simulink model "BumplessPID_UuT_Harness1"  (R2020a)
settings: Solver=ode8  StartTime=0.0  StopTime=40  FixedStep=0.1  RelTol=1e-3
settings Model: PauseTimes=12  Creator=Christian  LastModifiedBy=Christian

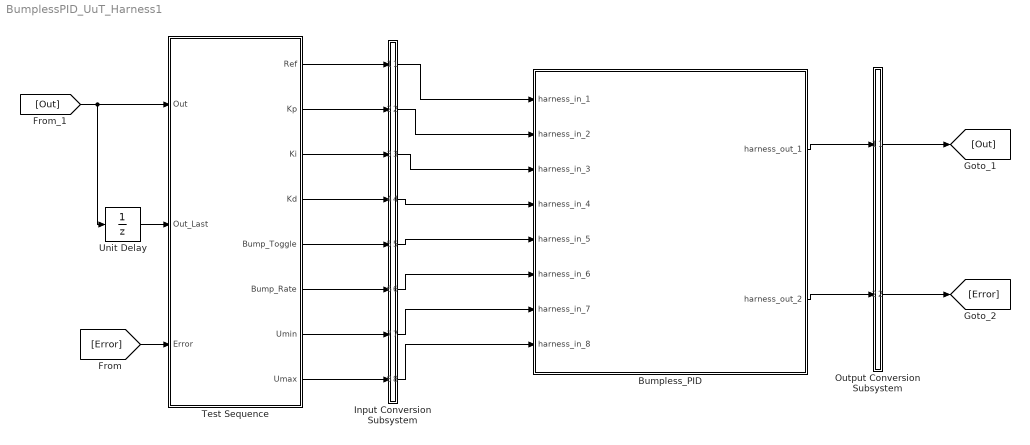
== system BumplessPID_UuT_Harness1 ==
  Bumpless_PID : Subsystem  Tag=__SL_testing_harness_stub_
  Input Conversion Subsystem : Subsystem  Tag=__SLT_ICS__  Description=|
      | Signal spec.
      | and routing
      settings: AttributesFormatString=%<Description>
  Output Conversion Subsystem : Subsystem  Tag=__SLT_OCS__  Description=|
      | Signal spec.
      | and routing
      settings: AttributesFormatString=%<Description>
  Test Sequence : Test Sequence  TreatAsAtomicUnit=on
  Unit Delay : UnitDelay  SampleTime=-1  HasFrameUpgradeWarning=on
  wires:
  Test Sequence/1(Ref) -> Input Conversion Subsystem/1(Inport_1)
  Test Sequence/2(Kp) -> Input Conversion Subsystem/2(Inport_2)
  Test Sequence/3(Ki) -> Input Conversion Subsystem/3(Inport_3)
  Test Sequence/4(Kd) -> Input Conversion Subsystem/4(Inport_4)
  Test Sequence/5(Bump_Toggle) -> Input Conversion Subsystem/5(Inport_5)
  Test Sequence/6(Bump_Rate) -> Input Conversion Subsystem/6(Inport_6)
  [Out] -> Unit Delay/1, Test Sequence/1(Out)
  Output Conversion Subsystem/1(Outport_1) -> [Out]
  Output Conversion Subsystem/2(Outport_2) -> [Error]
  [Error] -> Test Sequence/3(Error)
  Bumpless_PID/1(harness_out_1) -> Output Conversion Subsystem/1(Inport_1)
  Bumpless_PID/2(harness_out_2) -> Output Conversion Subsystem/2(Inport_2)
  Input Conversion Subsystem/1(Outport_1) -> Bumpless_PID/1(harness_in_1)
  Input Conversion Subsystem/2(Outport_2) -> Bumpless_PID/2(harness_in_2)
  Input Conversion Subsystem/3(Outport_3) -> Bumpless_PID/3(harness_in_3)
  Input Conversion Subsystem/4(Outport_4) -> Bumpless_PID/4(harness_in_4)
  Input Conversion Subsystem/5(Outport_5) -> Bumpless_PID/5(harness_in_5)
  Input Conversion Subsystem/6(Outport_6) -> Bumpless_PID/6(harness_in_6)
  Input Conversion Subsystem/7(Outport_7) -> Bumpless_PID/7(harness_in_7)
  Input Conversion Subsystem/8(Outport_8) -> Bumpless_PID/8(harness_in_8)
  Test Sequence/7(Umin) -> Input Conversion Subsystem/7(Inport_7)
  Test Sequence/8(Umax) -> Input Conversion Subsystem/8(Inport_8)
  Unit Delay/1 -> Test Sequence/2(Out_Last)

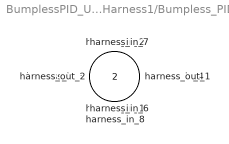
== system BumplessPID_UuT_Harness1/Bumpless_PID ==
  harness_in_1 : Inport
  harness_in_2 : Inport  Port=2
  harness_in_3 : Inport  Port=3
  harness_in_4 : Inport  Port=4
  harness_in_5 : Inport  Port=5
  harness_in_6 : Inport  Port=6
  harness_in_7 : Inport  Port=7
  harness_in_8 : Inport  Port=8
  harness_out_1 : Outport
  harness_out_2 : Outport  Port=2

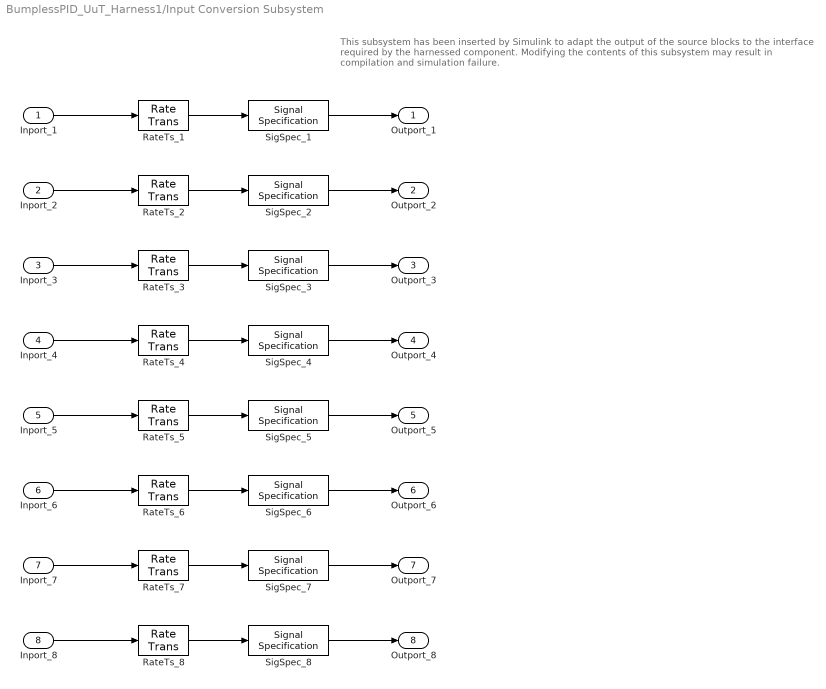
== system BumplessPID_UuT_Harness1/Input Conversion Subsystem ==
  note: This subsystem has been inserted by Simulink to adapt the output of the source blocks to the interface required by the harnessed component.
      |  Modifying the contents of this subsystem may result in compilation and simulation failure.
  Inport_1 : Inport
  Inport_2 : Inport  Port=2
  Inport_3 : Inport  Port=3
  Inport_4 : Inport  Port=4
  Inport_5 : Inport  Port=5
  Inport_6 : Inport  Port=6
  Inport_7 : Inport  Port=7
  Inport_8 : Inport  Port=8
  RateTs_{1..8} (8 alike) : RateTransition  OutPortSampleTime=[-1, 0]
  SigSpec_{1..6} (6 alike) : SignalSpecification  OutDataTypeStr=double  Dimensions=[1]  SampleTime=[-1, 0]
  SigSpec_7 : SignalSpecification  OutDataTypeStr=double  Dimensions=[1]
  SigSpec_8 : SignalSpecification  OutDataTypeStr=double  Dimensions=[1]
  Outport_1 : Outport
  Outport_2 : Outport  Port=2
  Outport_3 : Outport  Port=3
  Outport_4 : Outport  Port=4
  Outport_5 : Outport  Port=5
  Outport_6 : Outport  Port=6
  Outport_7 : Outport  Port=7
  Outport_8 : Outport  Port=8
  wires:
  SigSpec_1/1 -> Outport_1/1
  RateTs_1/1 -> SigSpec_1/1
  Inport_1/1 -> RateTs_1/1
  SigSpec_2/1 -> Outport_2/1
  RateTs_2/1 -> SigSpec_2/1
  Inport_2/1 -> RateTs_2/1
  SigSpec_3/1 -> Outport_3/1
  RateTs_3/1 -> SigSpec_3/1
  Inport_3/1 -> RateTs_3/1
  SigSpec_4/1 -> Outport_4/1
  RateTs_4/1 -> SigSpec_4/1
  Inport_4/1 -> RateTs_4/1
  SigSpec_5/1 -> Outport_5/1
  RateTs_5/1 -> SigSpec_5/1
  Inport_5/1 -> RateTs_5/1
  SigSpec_6/1 -> Outport_6/1
  RateTs_6/1 -> SigSpec_6/1
  Inport_6/1 -> RateTs_6/1
  SigSpec_7/1 -> Outport_7/1
  RateTs_7/1 -> SigSpec_7/1
  Inport_7/1 -> RateTs_7/1
  SigSpec_8/1 -> Outport_8/1
  RateTs_8/1 -> SigSpec_8/1
  Inport_8/1 -> RateTs_8/1

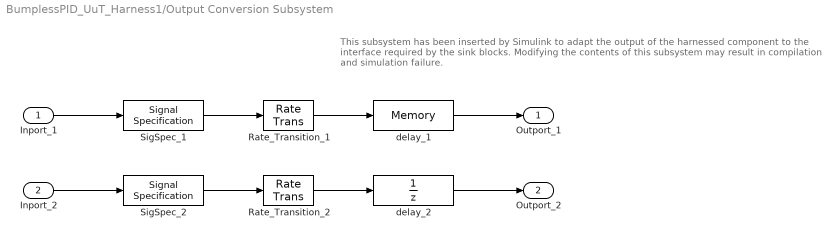
== system BumplessPID_UuT_Harness1/Output Conversion Subsystem ==
  note: This subsystem has been inserted by Simulink to adapt the output of the harnessed component to the interface required by the sink blocks.
      |  Modifying the contents of this subsystem may result in compilation and simulation failure.
  Inport_1 : Inport
  Inport_2 : Inport  Port=2
  Rate_Transition_1 : RateTransition  OutPortSampleTimeOpt=Inherit
  Rate_Transition_2 : RateTransition  OutPortSampleTimeOpt=Inherit
  SigSpec_1 : SignalSpecification  OutDataTypeStr=double  Dimensions=[1]
  SigSpec_2 : SignalSpecification  OutDataTypeStr=double  Dimensions=[1]  SampleTime=0.1
  delay_1 : Memory
  delay_2 : UnitDelay  SampleTime=-1
  Outport_1 : Outport
  Outport_2 : Outport  Port=2
  wires:
  Inport_1/1 -> SigSpec_1/1
  SigSpec_1/1 -> Rate_Transition_1/1
  Rate_Transition_1/1 -> delay_1/1
  delay_1/1 -> Outport_1/1
  Inport_2/1 -> SigSpec_2/1
  SigSpec_2/1 -> Rate_Transition_2/1
  Rate_Transition_2/1 -> delay_2/1
  delay_2/1 -> Outport_2/1

== stateflow chart BumplessPID_UuT_Harness1/Test Sequence ==
  settings: updateMethod=DISCRETE  sampleTime=0.1  stateMachineType=SIMPLIFIED_MACHINE
  state InitParams
    %% Initialize data outputs.
    Ref = 5;
    Kp = 0.1;
    Ki = 1;
    Kd = 0.01;
    Bump_Toggle = 1;
    Bump_Rate = 1;
    Umin = 0;
    Umax = 100;
  state Run
    Ref = 2;
    state BumplessOn
      verify(abs(Out-Out_Last) < Bump_Rate) % Check that output is bumpless
      Bump_Toggle = 0;
    state BumplessOff
      Bump_Toggle = 1;
    (default) -> (junction 35)
    Run -> (junction 35) [order 1]
    (junction 35) -> (junction 36) [order 1] : [Bump_Toggle == 1
        | ]
    (junction 36) -> BumplessOn [order 1] : [~in(BumplessOn)]
    (junction 36) -> (junction 39) [order 2]
    (junction 46) -> (junction 47)
    (junction 47) -> BumplessOff [order 1] : [~in(BumplessOff)]
    (junction 47) -> (junction 50) [order 2]
    (junction 35) -> (junction 46) [order 2]
  state Check_Lims
    verify(Umin <= Out <= Umax)
  (default) -> InitParams
  InitParams -> Run : [
      | after(10,sec)
      | ]
  Run -> Check_Lims [order 1] : [
      | after(10,sec)
      | ]
  data: Out input double size=[1]; Out_Last input; Ref output double size=[1]; Kp output double size=[1]; Ki output double size=[1]; Kd output double size=[1]; Bump_Toggle output double size=[1]; Bump_Rate output double size=[1]; Error input; Umin output; Umax output; CheckLims local
